simulink model "alpha"  (R2020a)
settings: Solver=VariableStepAuto  StartTime=0.0  StopTime=10  RelTol=1e-3
settings Model: Creator=User  LastModifiedBy=Nazwa Najmuddin
settings DataIOCC: ReturnWorkspaceOutputs=off  Refine=10

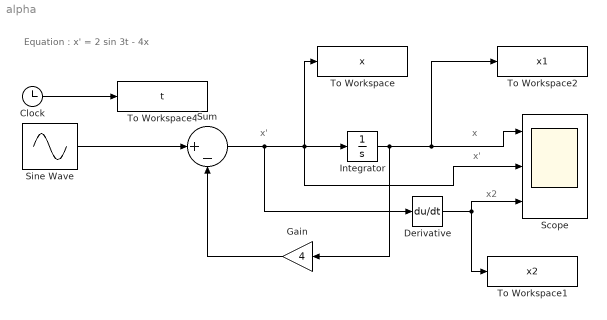
== system alpha ==
  note: x
  note: Equation :
      |  x' = 2 sin 3t - 4x
  note: x'
  note: x'
  note: x2
  Clock : Clock
  Derivative : Derivative
  Gain : Gain  Gain=4
  Integrator : Integrator
  Scope : Scope  NumInputPorts=3
  Sine Wave : Sin  Amplitude=2  Frequency=3  SampleTime=0
  Sum : Sum  Inputs=|+-
  To Workspace : ToWorkspace  VariableName=x  SampleTime=-1
  To Workspace1 : ToWorkspace  VariableName=x2  SampleTime=-1
  To Workspace2 : ToWorkspace  VariableName=x1  SampleTime=-1
  To Workspace4 : ToWorkspace  VariableName=t  SampleTime=-1
  wires:
  Clock/1 -> To Workspace4/1
  Sine Wave/1 -> Sum/1
  Integrator/1 -> To Workspace2/1, Scope/1, Gain/1
  Gain/1 -> Sum/2
  Sum/1 -> Derivative/1, Integrator/1, To Workspace/1, Scope/2
  Derivative/1 -> Scope/3, To Workspace1/1
